simulink model "prac222"  (R2022b)
settings: Solver=VariableStepAuto  StartTime=0.0  StopTime=100  RelTol=1e-3
settings Model: Creator=ESTHER  LastModifiedBy=ESTHER

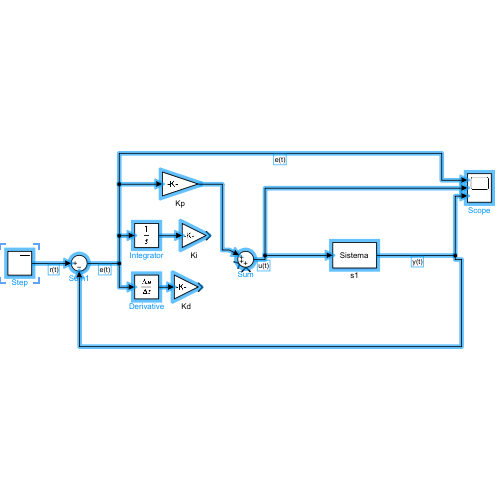
[thumbnail: Simulink's stored preview of the top-level diagram]
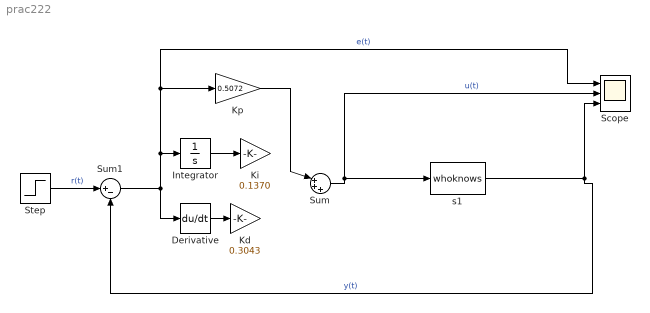
== system prac222 ==
  Derivative : Derivative
  Integrator : Integrator
  Kd : Gain  Gain=0.3043
  Ki : Gain  Gain=0.1370
  Kp : Gain  Gain=0.5072
  Scope : Scope  NumInputPorts=3
  Step : Step  SampleTime=0
  Sum : Sum  Inputs=|+++
  Sum1 : Sum  Inputs=|+-
  s1 : M-S-Function  FunctionName=whoknows  Parameters=L, P1, P2, T, R  mask{L=6, P1=1, P2=3, T=2, R=0}
      mask prompts: L "Laboratorio"; P1 "Primer digito del Puesto"; P2 "Segundo digito del Puesto"; T "Tipo de Planta"; R "Ruido"
      mask Display: disp('Sistema')
  wires:
  Kp/1 -> Sum/1
  Derivative/1 -> Kd/1
  Sum1/1 -> Integrator/1, Scope/1, Kp/1, Derivative/1  "e(t)"
  Step/1 -> Sum1/1  "r(t)"
  Integrator/1 -> Ki/1
  s1/1 -> Sum1/2, Scope/3  "y(t)"
  Sum/1 -> s1/1, Scope/2  "u(t)"
